simulink model "PVArrayGrid"  (R2024b)
settings: Solver=FixedStepDiscrete  StartTime=0.0  StopTime=2.5  RelTol=1e-3
PreLoadFcn:
  | Ts_Power=1e-6;
  | Ts_Control=100e-6;
InitFcn:
  | Ts_Power=1e-6;
  | Ts_Control=100e-6;
undefined symbols (not defined in the file): D1, Delta, DiscIntNeverNeededParam
libraries: spsSeriesRLCBranchLib x5, spsMeanLib x3, spsThreePhaseTransformerTwoWindingsLib x2, spsDistributedParametersLineLib x2, spsThreePhaseParallelRLCLoadLib x2, spsFourierLib x2, slpidlib x2, spsabctodq0Lib x2, spsVoltageMeasurementLib x2, spsThreePhaseSeriesRLCLoadLib x1, spsThreeLevelBridgeLib x1, spsThreePhaseSourceLib x1
(part 1 of 2)
settings Model: SimulationMode=accelerator  Creator=The MathWorks, Inc.  LastModifiedBy=chang
settings SolverCC: AlgebraicLoopSolver=TrustRegion
settings DataIOCC: LimitDataPoints=on  SaveFormat=Array  SignalLogging=off  DSMLogging=off  ReturnWorkspaceOutputs=off
settings OptimizationCC: ExpressionDepthLimit=2147483647  EfficientMapNaN2IntZero=off  LifeSpan=inf
settings DebuggingCC: UnderspecifiedInitializationDetection=Classic  MergeDetectMultiDrivingBlocksExec=none  SolverPrmCheckMsg=warning  FcnCallInpInsideContextMsg=warning  UnconnectedInputMsg=warning  UnconnectedOutputMsg=warning  UnconnectedLineMsg=warning  StateNameClashWarn=warning  SubsystemReferenceDiagnosticForUnitTest=warning  SFUnexpectedBacktrackingDiag=warning  SFNoUnconditionalDefaultTransitionDiag=warning  SFExecutionAtInitializationDiag=none  ArithmeticOperatorsInVariantConditions=warning
settings HardwareCC: ProdBitPerPointer=32  ProdBitPerSizeT=32  ProdBitPerPtrDiffT=32  ProdLargestAtomicFloat=None  ProdIntDivRoundTo=Undefined  ProdEndianess=Unspecified  ProdWordSize=32  ProdHWDeviceType=32-bit Generic  TargetBitPerPointer=64  TargetBitPerSizeT=64  TargetBitPerPtrDiffT=64  TargetLongLongMode=on  TargetIntDivRoundTo=Zero  TargetEndianess=LittleEndian  TargetWordSize=64  TargetHWDeviceType=MATLAB Host  ProdEqTarget=off
settings ModelReferenceCC: EnableRefExpFcnMdlSchedulingChecks=on  PropagateSignalLabelsOutOfModel=off
settings SFSimCC: SimUseLocalCustomCode=off  CustomCodeUndefinedFunction=UseInterfaceOnly
settings RTWCC: GPUComputeCapability=3.5
settings CodeAppCC: MaxIdLength=128
settings GRTTargetCC: TargetLangStandard=C89/C90 (ANSI)  CombineOutputUpdateFcns=off  GRTInterface=on
settings ConfigComp: CovMetricSettings=dw  CovSaveCumulativeToWorkspaceVar=on  CovSaveSingleToWorkspaceVar=on  CovExternalEMLEnable=off  CovSFcnEnable=off
settings SimscapeCC: SimscapeNormalizeSystem=off

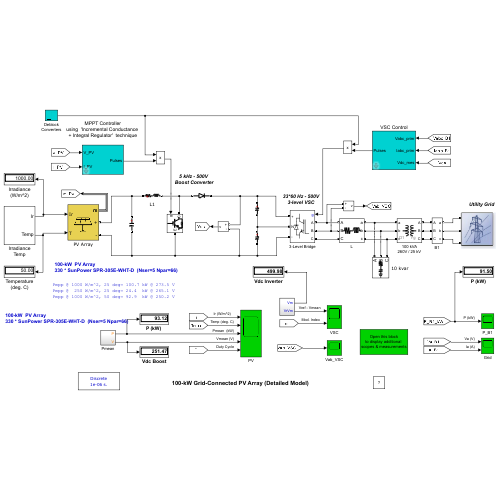
[thumbnail: Simulink's stored preview of the top-level diagram]
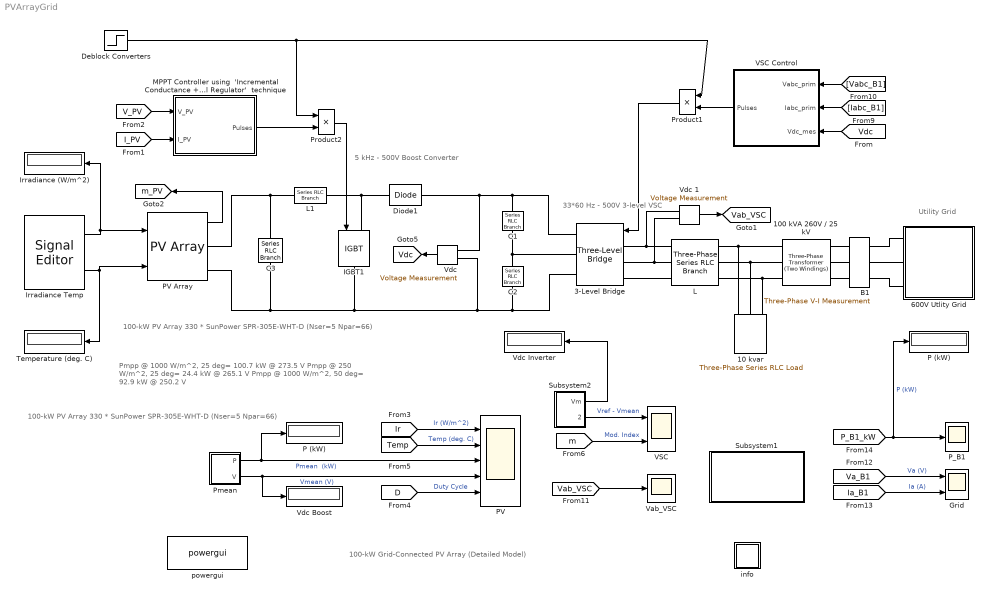
== system PVArrayGrid ==
  note: 5 kHz - 500V
      | Boost Converter
  note: 33*60 Hz - 500V
      | 3-level VSC
  note: 100-kW Grid-Connected PV Array (Detailed Model)
  note: Utility Grid
  note: Pmpp @ 1000 W/m^2, 25 deg= 100.7 kW @ 273.5 V
      | Pmpp @  250 W/m^2, 25 deg= 24.4  kW @ 265.1 V
      | Pmpp @ 1000 W/m^2, 50 deg= 92.9  kW @ 250.2 V
  note: 100-kW  PV Array
      | 330 * SunPower SPR-305E-WHT-D  (Nser=5 Npar=66)
  note: 100-kW  PV Array
      | 330 * SunPower SPR-305E-WHT-D  (Nser=5 Npar=66)
  10 kvar : spsThreePhaseSeriesRLCLoadLib/Three-Phase Series RLC Load  LConnTagsString=A|B|C  Configuration=Y (grounded)  NominalVoltage=240  Vabc=[1e3 1e3 1e3]  Vabcp=[1e3 1e3 1e3]  NominalFrequency=60  UnbalancedPower=off  ActivePower=10e3/100  InductivePower=0  CapacitivePower=10e3  Pabc=[10e3 9e3 11e3]  QLabc=[100 90 110]  QCabc=[100 90 110]  Pabcp=[10e3 9e3 11e3]  QLabcp=[100 90 110]  QCabcp=[100 90 110]  Measurements=None  LoadType=constant Z
  100 kVA 260V / 25 kV : spsThreePhaseTransformerTwoWindingsLib/Three-Phase Transformer (Two Windings)  Winding1Connection=Yg  Winding2Connection=Delta (D1)  CoreType=Three single-phase transformers  SetSaturation=off  Hysteresis=off  DataFile='hysteresis'  SetInitialFlux=off  Measurements=None  UNITS=pu  NominalPower=[100e3 , 60 ]  Winding1=[ 25e3 , 0.001 , 0.03 ]  Winding2=[ 260 , 0.001 , 0.03 ]  Rm=500  Lm=500  L0=0.5  Saturation=[ 0,0 ; 0.0024,1.2 ; 1.0,1.52 ]  InitialFluxes=[ 0.8 , -0.8 , 0.7 ]  BreakLoop=off  DiscreteSolver=Trapezoidal iterative  DataType=off  TransfoNumber=0
  3-Level Bridge : spsThreeLevelBridgeLib/Three-Level Bridge  Arms=3  SnubberResistance=1e6  SbubberCapacitance=inf  Device=IGBT / Diodes  Ron=0.2e-3  ForwardVoltages="[  0  0 ]"  Measurements=None
      settings: AttributesFormatString=\n
  600V Utlity Grid : Subsystem
      mask Display: image('$imagefile')
  B1 : spsThreePhaseVIMeasurementLib/Three-Phase V-I Measurement  VoltageMeasurement=phase-to-ground  SetLabelV=on  LabelV=Vabc_B1  Vpu=off  VpuLL=off  CurrentMeasurement=yes  SetLabelI=on  LabelI=Iabc_B1  Ipu=off  Pbase=100e6  Vbase=500e3  OutputType=Magnitude  PhasorSimulation=off  PSBequivalent=0
  C1 : spsSeriesRLCBranchLib/Series RLC Branch  LConnTagsString=__new0  RConnTagsString=__new0  BranchType=C  Resistance=1.0  Inductance=1.0  SetiL0=off  InitialCurrent=0  Capacitance=12000e-06  Setx0=off  InitialVoltage=0  Measurements=None
  C2 : spsSeriesRLCBranchLib/Series RLC Branch  LConnTagsString=__new0  RConnTagsString=__new0  BranchType=C  Resistance=1.0  Inductance=1.0  SetiL0=off  InitialCurrent=0  Capacitance=12000e-06  Setx0=off  InitialVoltage=0  Measurements=None
  C3 : spsSeriesRLCBranchLib/Series RLC Branch  LConnTagsString=__new0  RConnTagsString=__new0  BranchType=C  Resistance=1.0  Inductance=1.0  SetiL0=off  InitialCurrent=0  Capacitance=100e-6  Setx0=off  InitialVoltage=0  Measurements=Branch voltage
  Deblock Converters : Step  Time=0.05  SampleTime=0
  Diode1 : spsDiodeLib/Diode  Ron=1e-4  Lon=0  Vf=0  IC=0  UseSnubber=off  Rs=inf  Cs=inf  Measurements=off
  Grid : Scope  NumInputPorts=2
  IGBT1 : spsIGBTLib/IGBT  Ron=0.001  Lon=0  Vf=0  Tf=0  Tt=0  IC=0  Rs=1e5  Cs=inf  Measurements=off
  Irradiance (W/m^2) : Display
      settings: Format=bank  Decimation=1000
  Irradiance Temp : SignalEditorBlockLib/Signal Editor  FileName=PVArrayGridData.mat  ActiveScenario=Ramp_up_down_Irradiance  ActiveSignal=Temp  IsBus=off  OutputBusObjectStr=Bus: BusObject  SampleTime=0  OutputAfterFinalValue=Extrapolation  Unit=inherit  PreserveSignalName=on  ApplySigPropsToAllScenarios=on  ApplySigPropsToAllSignals=off
  L : spsThreePhaseSeriesRLCBranchLib/Three-Phase Series RLC Branch  LConnTagsString=A|B|C  RConnTagsString=A|B|C  BranchType=RL  Resistance=500e-6*377/50/2  Inductance=500e-6/2  Capacitance=inf  Measurements=None
  L1 : spsSeriesRLCBranchLib/Series RLC Branch  LConnTagsString=__new0  RConnTagsString=__new0  BranchType=RL  Resistance=0.005  Inductance=5e-3  SetiL0=off  InitialCurrent=0  Capacitance=1e-6  Setx0=off  InitialVoltage=0  Measurements=None
  "MPPT Controller using  'Incremental Conductance + Integral Regulator'  technique " : Subsystem  mask(Boost Control - MPPT){fc=5000, T_MPPT=200e-6, Dinit=0.5}
      mask prompts: fc "PWM switching frequency (Hz)"; T_MPPT "Time window used by MPPT control (s)"; Dinit "Initial value of duty cycle"
  P (kW) : Display
      settings: Format=bank  Decimation=2000
  "P (kW) " : Display
      settings: Format=bank  Decimation=2000
  PV : Scope  NumInputPorts=5
  PV Array : spsPVArrayLib/PV Array  Npar=66  Nser=5  PlotType=array @ 1000 W/m2 & specified temperatures  S_vec="[ 1000  250 ]"  Temp_C_vec="[0 25 50  ]"  ModuleName=SunPower SPR-305E-WHT-D  PlotWhenSelected=off  Pm=305.226  Ncell=96  Voc=64.2  Isc=5.96  Vm=54.7  Im=5.58  beta_Voc_pc=-0.2727  alpha_Isc_pc=0.061745  beta_Voc=-0.17507  alpha_Isc=0.00368  IL=5.9657  I0=6.3076e-12  nI=0.94489  Rsh=393.2054  Rs=0.37428  RobustModel=off  RobustCellTemperature=25  BAL=on  Tc=1e-6  Tfilter=5e-5
  P_B1 : Scope
  Pmean : Subsystem
  Product1 : Product  RndMeth=Zero
  Product2 : Product  RndMeth=Zero
  Subsystem1 : Subsystem
      mask Display: disp('Open this block\nto display additional \nscopes & measurements')
  Subsystem2 : Subsystem
  Temperature (deg. C) : Display
      settings: Format=bank  Decimation=1000
  VSC : Scope  NumInputPorts=2
  VSC Control : Subsystem  mask(VSC Main Controller){nom=[ 100e3  60 ], Vnom=[ 25e3 260 ], Vnom_dc=500, RLxfo=[0.002  0.06 ], RLchoke=[2e-3  250e-6  ], K_VDCreg=[7  800], K_Ireg=[0.3 20], Ts=Ts_Control}
      mask prompts: nom "Nominal power and frequency [ Pnom(VA)  Fnom(Hz) ]:"; Vnom "Nominal primary and secondary voltages (Vrms LL) [ Vnom_prim   Vnom_sec ]:"; Vnom_dc "Nominal DC bus voltage (V):"; RLxfo "Total transformer leakage impedance (pu/Pnom) [ Rxfo  Lxf ]"; RLchoke "Choke impedance [ R(ohm) L(H) ]"; K_VDCreg "VDC regultator gains [ Kp  Ki ]:"; K_Ireg "Current regulator gains [ Kp  Ki ]:"; Ts "Sample time"
      mask init:
      | Pnom=nom(1);
      | Fnom=nom(2);
      | Vnom_prim=Vnom(1);
      | Vnom_sec=Vnom(2);
      | Zbase=Vnom_sec^2/Pnom;
      | Rtot_pu=RLxfo(1) + RLchoke(1)/Zbase;
      | Ltot_pu=RLxfo(2) + RLchoke(2)/(Zbase/(2*pi*Fnom));
      | Kp_VDCreg=K_VDCreg(1);
      | Ki_VDCreg=K_VDCreg(2);
      | Kp_Ireg=K_Ireg(1);
      | Ki_Ireg=K_Ireg(2);
      | Vdc_ref=Vnom_dc;
      | % Used to determine initial value of Boost Control (MPPT)
      | assignin('base','Vdc_ref_Inv',Vdc_ref);
  Vab_VSC : Scope
  "Vdc " : spsVoltageMeasurementLib/Voltage Measurement  Tag=PoWeRsYsTeMmEaSuReMeNt  PhasorSimulation=off  OutputType=Magnitude  PSBequivalent=0
  Vdc 1 : spsVoltageMeasurementLib/Voltage Measurement  Tag=PoWeRsYsTeMmEaSuReMeNt  PhasorSimulation=off  OutputType=Magnitude  PSBequivalent=0
  Vdc Boost : Display
      settings: Format=bank  Decimation=2000
  Vdc Inverter : Display
      settings: Format=bank  Decimation=2000
  info : Subsystem
      settings: OpenFcn="showExample(\"simscapeelectricalsps/PVArrayGridExample\")"
      mask Display: disp('?')
  powergui : spspowerguiLib/powergui  Priority=1  SimulationMode=Discrete  SampleTime=Ts_Power  frequency=60  Iterations=50  frequencyindice=0  Pbase=100e6  ErrMax=1e-4  UnitsV=kV  UnitsW=MW  buscounter=0  FunctionMessages=off  echomessages=off  EnableUseOfTLC=off  CurrentSourceSwitches=off  DisableSnubberDevices=off  DisableRonSwitches=off  DisableVfSwitches=off  DisplayEquations=off  AutomaticDiscreteSolvers=off  SolverType=Tustin/Backward Euler (TBE)  Interpol=off  ExternalGateDelay=off  methode=off  Ts=0  x0status=blocks  SPID=off  SwTol=0  HookPort=off  NonlinearTolerance=1e-8  nMaxIteration=10  ContinueOnMaxIteration=off  RestoreLinks=warning  ResistiveCurrentMeasurement=off  Frange=[0:2:500]  Ylog=off  Xlog=on  ShowGrid=off  save=off  variable=ZData  structure=0  ZoomFFT=on  StartTime=0.0  cycles=1  DisplayStyle=1  fundamental=60  FreqAxis=off  MaxFrequency=1000  frequencyindicesteady=1  RmsSteady=1  display=off
  tag scope: Vab_VSC=global, Vdc=global, m_PV=global
  wires:
  "Vdc "/1 -> [Vdc]
  Product2/1 -> IGBT1/1
  "MPPT Controller using  'Incremental Conductance + Integral Regulator'  technique "/1(Pulses) -> Product2/2
  Deblock Converters/1 -> Product1/1, Product2/1
  [Vabc_B1] -> VSC Control/1(Vabc_prim)
  [Iabc_B1] -> VSC Control/2(Iabc_prim)
  [Vdc] -> VSC Control/3(Vdc_mes)
  VSC Control/1(Pulses) -> Product1/2
  Product1/1 -> 3-Level Bridge/1
  [I_PV] -> "MPPT Controller using  'Incremental Conductance + Integral Regulator'  technique "/2(I_PV)
  [V_PV] -> "MPPT Controller using  'Incremental Conductance + Integral Regulator'  technique "/1(V_PV)
  Pmean/1(P) -> "P (kW) "/1, PV/3  "Pmean  (kW)"
  [m] -> VSC/2  "Mod. Index"
  Vdc 1/1 -> [Vab_VSC]
  [Vab_VSC] -> Vab_VSC/1
  [Ia_B1] -> Grid/2  "Ia (A)"
  [Va_B1] -> Grid/1  "Va (V)"
  [P_B1_kW] -> P_B1/1, P (kW)/1  "P (kW)"
  Pmean/2(V) -> Vdc Boost/1, PV/4  "Vmean (V)"
  Subsystem2/2(VrVm) -> VSC/1  "Vref - Vmean"
  Subsystem2/1(Vm) -> Vdc Inverter/1
  PV Array/1 -> [m_PV]
  Irradiance Temp/1 -> PV Array/1, Irradiance (W/m^2)/1
  Irradiance Temp/2 -> PV Array/2, Temperature (deg. C)/1
  [D] -> PV/5  "Duty Cycle"
  [Temp] -> PV/2  "Temp (deg. C)"
  [Ir] -> PV/1  "Ir (W/m^2)"
  connections:
  3-Level Bridge/RConn1 -- Diode1/RConn1 -- "Vdc "/LConn1 -- C1/LConn1
  L1/RConn1 -- Diode1/LConn1 -- IGBT1/LConn1
  3-Level Bridge/RConn3 -- C2/RConn1 -- "Vdc "/LConn2 -- IGBT1/RConn1 -- PV Array/RConn2 -- C3/RConn1
  3-Level Bridge/LConn1 -- L/LConn1 -- Vdc 1/LConn1
  3-Level Bridge/LConn2 -- L/LConn2 -- Vdc 1/LConn2
  3-Level Bridge/LConn3 -- L/LConn3
  L/RConn1 -- 100 kVA 260V / 25 kV/RConn1 -- 10 kvar/LConn1
  L/RConn2 -- 100 kVA 260V / 25 kV/RConn2 -- 10 kvar/LConn2
  L/RConn3 -- 100 kVA 260V / 25 kV/RConn3 -- 10 kvar/LConn3
  B1/LConn1 -- 100 kVA 260V / 25 kV/LConn1
  B1/LConn2 -- 100 kVA 260V / 25 kV/LConn2
  B1/LConn3 -- 100 kVA 260V / 25 kV/LConn3
  C2/LConn1 -- C1/RConn1 -- 3-Level Bridge/RConn2
  C3/LConn1 -- PV Array/RConn1 -- L1/LConn1
  B1/RConn2 -- 600V Utlity Grid/LConn2
  B1/RConn1 -- 600V Utlity Grid/LConn1
  B1/RConn3 -- 600V Utlity Grid/LConn3

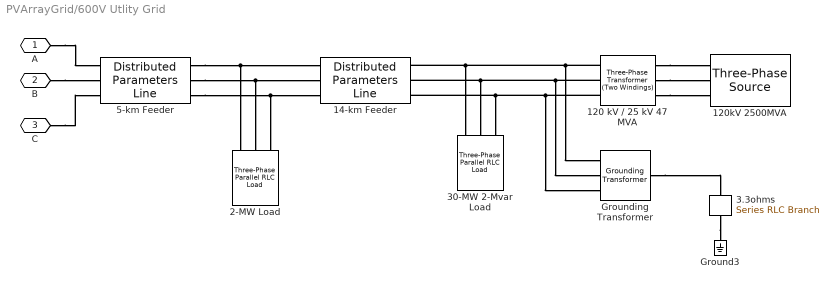
== system PVArrayGrid/600V Utlity Grid ==
  120 kV / 25 kV 47 MVA : spsThreePhaseTransformerTwoWindingsLib/Three-Phase Transformer (Two Windings)  Winding1Connection=Yg  Winding2Connection=Delta (D1)  CoreType=Three single-phase transformers  SetSaturation=off  Hysteresis=off  DataFile='basic_model'  SetInitialFlux=off  Measurements=None  UNITS=pu  NominalPower=[47e6 60 ]  Winding1="[ 120e3  0.08/30   0.08 ]"  Winding2="[ 25e3  0.08/30  0.08]"  Rm=500  Lm=500  L0=0.5  Saturation="[ 0,0  ;  0.005,1.2  ;  1.0,1.4 ]"  InitialFluxes=[ 0.8 , -0.8 , 0.7 ]  BreakLoop=off  DiscreteSolver=Trapezoidal iterative  DataType=off  TransfoNumber=0
  120kV 2500MVA : spsThreePhaseSourceLib/Three-Phase Source  InternalConnection=Yg  VoltagePhases=off  Voltage=120e3  PhaseAngle=0  Voltage_phases=[25e3 25e3 25e3]/sqrt(3)  PhaseAngles_phases=[0 -120 +120]  Frequency=60  NonIdealSource=on  SpecifyImpedance=on  Resistance=0.8929  Inductance=16.58e-3  ShortCircuitLevel=2500e6  BaseVoltage=120e3  XRratio=7  BusType=swing  Pref=0  Qref=0  Prefabc=[10e3, 10e3, 10e3]  Qrefabc=[0, 0, 0]  Qmin=-inf  Qmax=inf
  14-km Feeder : spsDistributedParametersLineLib/Distributed Parameters Line  Phases=3  Length=14  Frequency=60  Resistance=[0.1153 0.413]  Inductance=[1.05e-3 3.32e-3]  Capacitance=[11.33e-009 5.01e-009]  x1=[-5.8e-05 -2.72104735733765e-09 0 0;-5.7e-05 -2.72148457100924e-09 0 0;-5.6e-05 -2.72192139789718e-09 0 0;-5.5e-05 -2.72235783793939e-09 0 0;-5.4e-05 -2.72279389107383e-09 0 0;-5.3e-05 -2.72322955723854e-09 0 0;-5.2e-05 -2.7236648363716e-09 0 0;-5.1e-05 -2.72409972841114e-09 0 0;-5e-05 -2.72453423329536e-09 0 0;-4.9e-05 -2.7249683509625e-09 -3790.73535189766 -24061.4134200297;-4.8e-05 -2.72540208135087e-09 -3781.66414358226 -24062.8407837241;-4.7e-05 -2.72583542439882e-09 -3772.59239780806 -24064.2647275522;-4.6e-05 -2.72626838004477e-09 -3763.52011586433 -24065.6852513116;-4.5e-05 -2.72670094822718e-09 -3754.44729904047 -24067.1023548004;-4.4e-05 -2.72713312888457e-09 -3745.37394862591 -24068.5160378172;-4.3e-05 -2.72756492195553e-09 -3736.30006591019 -24069.9263001612;-4.2e-05 -2.72799632737868e-09 -3727.2256521829 -24071.3331416318;-4.1e-05 -2.72842734509272e-09 -3718.15070873373 -24072.7365620291;-4e-05 -2.72885797503638e-09 -3709.07523685241 -24074.1365611537;-3.9e-05 -2.72928821714846e-09 -3699.99923782879 -24075.5331388067;-3.8e-05 -2.72971807136783e-09 -3690.92271295276 -24076.9262947894;-3.7e-05 -2.73014753763337e-09 -3681.8456635143 -24078.3160289039;-3.6e-05 -2.73057661588407e-09 -3672.76809080346 -24079.7023409528;-3.5e-05 -2.73100530605893e-09 -3663.68999611036 -24081.0852307389;-3.4e-05 -2.73143360809703e-09 -3654.61138072521 -24082.4646980658;-3.3e-05 -2.7318615219375e-09 -3645.53224593827 -24083.8407427373;-3.2e-05 -2.73228904751952e-09 -3636.45259303991 -24085.213364558;-3.1e-05 -2.73271618478233e-09 -3627.37242332053 -24086.5825633327;-3e-05 -2.73314293366523e-09 -3618.29173807063 -24087.9483388669;-2.9e-05 -2.73356929410757e-09 -3609.21053858078 -24089.3106909664;-2.8e-05 -2.73399526604874e-09 -3600.12882614163 -24090.6696194376;-2.7e-05 -2.73442084942822e-09 -3591.04660204388 -24092.0251240874;-2.6e-05 -2.73484604418551e-09 -3581.96386757832 -24093.3772047232;-2.5e-05 -2.73527085026018e-09 -3572.88062403581 -24094.7258611527;-2.4e-05 -2.73569526759187e-09 -3563.79687270728 -24096.0710931843;-2.3e-05 -2.73611929612025e-09 -3554.71261488374 -24097.4129006268;-2.2e-05 -2.73654293578505e-09 -3545.62785185626 -24098.7512832896;-2.1e-05 -2.73696618652608e-09 -3536.54258491599 -24100.0862409823;-2e-05 -2.73738904828317e-09 -3527.45681535414 -24101.4177735154;-1.9e-05 -2.73781152099623e-09 -3518.37054446202 -24102.7458806994;-1.8e-05 -2.73823360460521e-09 -3509.28377353097 -24104.0705623458;-1.7e-05 -2.73865529905013e-09 -3500.19650385244 -24105.3918182661;-1.6e-05 -2.73907660427106e-09 -3491.10873671792 -24106.7096482727;-1.5e-05 -2.73949752020812e-09 -3482.020473419 -24108.0240521782;-1.4e-05 -2.73991804680148e-09 -3472.93171524731 -24109.3350297958;-1.3e-05 -2.74033818399138e-09 -3463.84246349457 -24110.6425809393;-1.2e-05 -2.74075793171812e-09 -3454.75271945257 -24111.9467054227;-1.1e-05 -2.74117728992202e-09 -3445.66248441316 -24113.2474030608;-1e-05 -2.74159625854351e-09 -3436.57175966826 -24114.5446736687;-9e-06 -2.74201483752302e-09 -3427.48054650988 -24115.8385170619;-8e-06 -2.74243302680107e-09 -3418.38884623008 -24117.1289330567;-7e-06 -2.74285082631822e-09 -3409.29666012098 -24118.4159214696;-6e-06 -2.74326823601511e-09 -3400.20398947479 -24119.6994821177;-5e-06 -2.7436852558324e-09 -3391.11083558379 -24120.9796148187;-4e-06 -2.74410188571082e-09 -3382.01719974031 -24122.2563193904;-3e-06 -2.74451812559117e-09 -3372.92308323676 -24123.5295956516;-2e-06 -2.74493397541429e-09 -3363.82848736562 -24124.7994434213;-1e-06 -2.74534943512107e-09 -3354.73341341943 -24126.0658625189]  x2=[-5.8e-05 -2.96070926633097e-09 0 0;-5.7e-05 -2.96113943631565e-09 0 0;-5.6e-05 -2.96156918545639e-09 0 0;-5.5e-05 -2.96199851369209e-09 0 0;-5.4e-05 -2.96242742096175e-09 0 0;-5.3e-05 -2.9628559072044e-09 0 0;-5.2e-05 -2.96328397235915e-09 0 0;-5.1e-05 -2.96371161636516e-09 0 0;-5e-05 -2.96413883916166e-09 0 0;-4.9e-05 -2.96456564068792e-09 -3379.39242591109 -24244.0512732198;-4.8e-05 -2.96499202088329e-09 -3370.25239397928 -24245.3235513097;-4.7e-05 -2.96541797968717e-09 -3361.11188305945 -24246.5923835984;-4.6e-05 -2.96584351703902e-09 -3351.97089445066 -24247.8577699056;-4.5e-05 -2.96626863287837e-09 -3342.82942945205 -24249.1197100514;-4.4e-05 -2.96669332714479e-09 -3333.68748936283 -24250.3782038566;-4.3e-05 -2.96711759977792e-09 -3324.54507548227 -24251.6332511421;-4.2e-05 -2.96754145071747e-09 -3315.40218910971 -24252.8848517298;-4.1e-05 -2.9679648799032e-09 -3306.25883154456 -24254.1330054416;-4e-05 -2.96838788727493e-09 -3297.1150040863 -24255.3777121002;-3.9e-05 -2.96881047277254e-09 -3287.97070803446 -24256.6189715286;-3.8e-05 -2.96923263633598e-09 -3278.82594468866 -24257.8567835506;-3.7e-05 -2.96965437790523e-09 -3269.68071534857 -24259.0911479901;-3.6e-05 -2.97007569742038e-09 -3260.53502131393 -24260.3220646718;-3.5e-05 -2.97049659482152e-09 -3251.38886388455 -24261.5495334206;-3.4e-05 -2.97091707004886e-09 -3242.24224436029 -24262.7735540622;-3.3e-05 -2.97133712304262e-09 -3233.09516404111 -24263.9941264226;-3.2e-05 -2.97175675374311e-09 -3223.947624227 -24265.2112503283;-3.1e-05 -2.97217596209069e-09 -3214.79962621804 -24266.4249256063;-3e-05 -2.97259474802578e-09 -3205.65117131435 -24267.6351520841;-2.9e-05 -2.97301311148887e-09 -3196.50226081614 -24268.8419295897;-2.8e-05 -2.97343105242049e-09 -3187.35289602367 -24270.0452579517;-2.7e-05 -2.97384857076124e-09 -3178.20307823727 -24271.245136999;-2.6e-05 -2.97426566645179e-09 -3169.05280875733 -24272.4415665611;-2.5e-05 -2.97468233943286e-09 -3159.90208888432 -24273.6345464679;-2.4e-05 -2.97509858964522e-09 -3150.75091991874 -24274.8240765499;-2.3e-05 -2.97551441702973e-09 -3141.5993031612 -24276.010156638;-2.2e-05 -2.97592982152728e-09 -3132.44723991233 -24277.1927865637;-2.1e-05 -2.97634480307883e-09 -3123.29473147284 -24278.3719661589;-2e-05 -2.97675936162541e-09 -3114.14177914353 -24279.547695256;-1.9e-05 -2.9771734971081e-09 -3104.98838422521 -24280.7199736878;-1.8e-05 -2.97758720946803e-09 -3095.8345480188 -24281.8888012879;-1.7e-05 -2.97800049864642e-09 -3086.68027182526 -24283.05417789;-1.6e-05 -2.97841336458453e-09 -3077.52555694561 -24284.2161033286;-1.5e-05 -2.97882580722367e-09 -3068.37040468094 -24285.3745774385;-1.4e-05 -2.97923782650523e-09 -3059.21481633242 -24286.529600055;-1.3e-05 -2.97964942237066e-09 -3050.05879320124 -24287.6811710141;-1.2e-05 -2.98006059476145e-09 -3040.90233658868 -24288.829290152;-1.1e-05 -2.98047134361916e-09 -3031.74544779609 -24289.9739573056;-1e-05 -2.98088166888544e-09 -3022.58812812485 -24291.1151723122;-9e-06 -2.98129157050194e-09 -3013.43037887644 -24292.2529350096;-8e-06 -2.98170104841043e-09 -3004.27220135236 -24293.387245236;-7e-06 -2.9821101025527e-09 -2995.1135968542 -24294.5181028304;-6e-06 -2.98251873287062e-09 -2985.9545666836 -24295.645507632;-5e-06 -2.98292693930612e-09 -2976.79511214227 -24296.7694594805;-4e-06 -2.98333472180117e-09 -2967.63523453196 -24297.8899582161;-3e-06 -2.98374208029782e-09 -2958.4749351545 -24299.0070036798;-2e-06 -2.98414901473818e-09 -2949.31421531178 -24300.1205957126;-1e-06 -2.98455552506442e-09 -2940.15307630573 -24301.2307341564]  x3=[-5.8e-05 -8.55897584940559e-12 0 0;-5.7e-05 -8.56403370536508e-12 0 0;-5.6e-05 -8.5690903441844e-12 0 0;-5.5e-05 -8.57414576514486e-12 0 0;-5.4e-05 -8.579199967528e-12 0 0;-5.3e-05 -8.5842529506155e-12 0 0;-5.2e-05 -8.5893047136892e-12 0 0;-5.1e-05 -8.59435525603115e-12 0 0;-5e-05 -8.59940457692354e-12 0 0;-4.9e-05 -8.60445267564877e-12 -23.544284738252 -155.681477773854;-4.8e-05 -8.60949955148938e-12 -23.4855925321333 -155.690342696974;-4.7e-05 -8.61454520372809e-12 -23.4268969881881 -155.699185493025;-4.6e-05 -8.61958963164782e-12 -23.3681981147585 -155.70800616075;-4.5e-05 -8.62463283453162e-12 -23.3094959201867 -155.716804698894;-4.4e-05 -8.62967481166275e-12 -23.2507904128157 -155.725581106208;-4.3e-05 -8.63471556232464e-12 -23.1920816009888 -155.734335381443;-4.2e-05 -8.63975508580088e-12 -23.13336949305 -155.743067523356;-4.1e-05 -8.64479338137524e-12 -23.0746540973434 -155.751777530706;-4e-05 -8.64983044833166e-12 -23.0159354222139 -155.760465402255;-3.9e-05 -8.65486628595427e-12 -22.9572134760066 -155.769131136768;-3.8e-05 -8.65990089352737e-12 -22.8984882670674 -155.777774733014;-3.7e-05 -8.66493427033542e-12 -22.8397598037422 -155.786396189764;-3.6e-05 -8.66996641566306e-12 -22.7810280943779 -155.794995505792;-3.5e-05 -8.67499732879512e-12 -22.7222931473214 -155.803572679878;-3.4e-05 -8.6800270090166e-12 -22.6635549709203 -155.8121277108;-3.3e-05 -8.68505545561266e-12 -22.6048135735226 -155.820660597345;-3.2e-05 -8.69008266786864e-12 -22.5460689634767 -155.829171338299;-3.1e-05 -8.69510864507008e-12 -22.4873211491317 -155.837659932452;-3e-05 -8.70013338650266e-12 -22.4285701388368 -155.846126378598;-2.9e-05 -8.70515689145226e-12 -22.3698159409419 -155.854570675534;-2.8e-05 -8.71017915920492e-12 -22.3110585637972 -155.86299282206;-2.7e-05 -8.71520018904688e-12 -22.2522980157536 -155.871392816978;-2.6e-05 -8.72021998026452e-12 -22.1935343051622 -155.879770659096;-2.5e-05 -8.72523853214443e-12 -22.1347674403745 -155.888126347221;-2.4e-05 -8.73025584397336e-12 -22.0759974297428 -155.896459880168;-2.3e-05 -8.73527191503823e-12 -22.0172242816195 -155.90477125675;-2.2e-05 -8.74028674462615e-12 -21.9584480043576 -155.913060475788;-2.1e-05 -8.74530033202441e-12 -21.8996686063106 -155.921327536102;-2e-05 -8.75031267652044e-12 -21.8408860958322 -155.929572436519;-1.9e-05 -8.7553237774019e-12 -21.7821004812769 -155.937795175866;-1.8e-05 -8.7603336339566e-12 -21.7233117709993 -155.945995752974;-1.7e-05 -8.76534224547251e-12 -21.6645199733546 -155.954174166679;-1.6e-05 -8.77034961123781e-12 -21.6057250966984 -155.962330415817;-1.5e-05 -8.77535573054084e-12 -21.5469271493869 -155.97046449923;-1.4e-05 -8.78036060267011e-12 -21.4881261397765 -155.978576415762;-1.3e-05 -8.78536422691433e-12 -21.4293220762242 -155.98666616426;-1.2e-05 -8.79036660256235e-12 -21.3705149670873 -155.994733743573;-1.1e-05 -8.79536772890325e-12 -21.3117048207236 -156.002779152556;-1e-05 -8.80036760522623e-12 -21.2528916454914 -156.010802390064;-9e-06 -8.80536623082072e-12 -21.1940754497493 -156.018803454959;-8e-06 -8.81036360497629e-12 -21.1352562418564 -156.026782346102;-7e-06 -8.81535972698271e-12 -21.0764340301722 -156.034739062359;-6e-06 -8.82035459612991e-12 -21.0176088230567 -156.0426736026;-5e-06 -8.82534821170802e-12 -20.9587806288703 -156.050585965698;-4e-06 -8.83034057300732e-12 -20.8999494559738 -156.058476150526;-3e-06 -8.8353316793183e-12 -20.8411153127283 -156.066344155965;-2e-06 -8.84032152993161e-12 -20.7822782074955 -156.074189980896;-1e-06 -8.84531012413806e-12 -20.7234381486375 -156.082013624204]  x4=[-5.8e-05 1.93112949511814e-12 0 0;-5.7e-05 1.93533782185214e-12 0 0;-5.6e-05 1.93954587353147e-12 0 0;-5.5e-05 1.94375364955807e-12 0 0;-5.4e-05 1.94796114933393e-12 0 0;-5.3e-05 1.95216837226107e-12 0 0;-5.2e-05 1.95637531774154e-12 0 0;-5.1e-05 1.96058198517746e-12 0 0;-5e-05 1.96478837397095e-12 0 0;-4.9e-05 1.96899448352419e-12 -1.35581366009174 -2.15298522698201;-4.8e-05 1.9732003132394e-12 -1.3550019074566 -2.1534962036844;-4.7e-05 1.97740586251885e-12 -1.35418996224548 -2.15400687432695;-4.6e-05 1.98161113076482e-12 -1.35337782457375 -2.15451723883709;-4.5e-05 1.98581611737966e-12 -1.35256549455686 -2.15502729714228;-4.4e-05 1.99002082176574e-12 -1.35175297231025 -2.15553704917003;-4.3e-05 1.99422524332548e-12 -1.35094025794939 -2.15604649484789;-4.2e-05 1.99842938146134e-12 -1.35012735158979 -2.15655563410346;-4.1e-05 2.00263323557581e-12 -1.34931425334699 -2.15706446686438;-4e-05 2.00683680507144e-12 -1.34850096333653 -2.15757299305833;-3.9e-05 2.01104008935081e-12 -1.34768748167402 -2.15808121261305;-3.8e-05 2.01524308781652e-12 -1.34687380847506 -2.15858912545629;-3.7e-05 2.01944579987126e-12 -1.3460599438553 -2.15909673151588;-3.6e-05 2.0236482249177e-12 -1.3452458879304 -2.15960403071968;-3.5e-05 2.02785036235861e-12 -1.34443164081605 -2.16011102299557;-3.4e-05 2.03205221159675e-12 -1.34361720262799 -2.16061770827152;-3.3e-05 2.03625377203495e-12 -1.34280257348195 -2.1611240864755;-3.2e-05 2.04045504307608e-12 -1.34198775349373 -2.16163015753556;-3.1e-05 2.04465602412305e-12 -1.34117274277912 -2.16213592137976;-3e-05 2.04885671457879e-12 -1.34035754145394 -2.16264137793623;-2.9e-05 2.0530571138463e-12 -1.33954214963407 -2.16314652713313;-2.8e-05 2.05725722132861e-12 -1.33872656743539 -2.16365136889866;-2.7e-05 2.06145703642879e-12 -1.33791079497381 -2.16415590316108;-2.6e-05 2.06565655854995e-12 -1.33709483236526 -2.16466012984869;-2.5e-05 2.06985578709525e-12 -1.33627867972572 -2.16516404888981;-2.4e-05 2.07405472146787e-12 -1.33546233717118 -2.16566766021284;-2.3e-05 2.07825336107107e-12 -1.33464580481765 -2.16617096374619;-2.2e-05 2.08245170530811e-12 -1.33382908278119 -2.16667395941834;-2.1e-05 2.08664975358233e-12 -1.33301217117788 -2.1671766471578;-2e-05 2.09084750529707e-12 -1.3321950701238 -2.16767902689313;-1.9e-05 2.09504495985576e-12 -1.3313777797351 -2.16818109855292;-1.8e-05 2.09924211666184e-12 -1.33056030012792 -2.16868286206583;-1.7e-05 2.10343897511879e-12 -1.32974263141845 -2.16918431736053;-1.6e-05 2.10763553463016e-12 -1.32892477372289 -2.16968546436577;-1.5e-05 2.11183179459951e-12 -1.32810672715749 -2.17018630301031;-1.4e-05 2.11602775443047e-12 -1.3272884918385 -2.17068683322299;-1.3e-05 2.1202234135267e-12 -1.32647006788222 -2.17118705493265;-1.2e-05 2.12441877129189e-12 -1.32565145540496 -2.17168696806821;-1.1e-05 2.12861382712979e-12 -1.32483265452306 -2.17218657255863;-1e-05 2.1328085804442e-12 -1.32401366535289 -2.17268586833288;-9e-06 2.13700303063895e-12 -1.32319448801086 -2.17318485532002;-8e-06 2.1411971771179e-12 -1.32237512261338 -2.17368353344913;-7e-06 2.14539101928499e-12 -1.3215555692769 -2.17418190264933;-6e-06 2.14958455654416e-12 -1.3207358281179 -2.17467996284979;-5e-06 2.15377778829943e-12 -1.31991589925289 -2.17517771397973;-4e-06 2.15797071395484e-12 -1.3190957827984 -2.17567515596841;-3e-06 2.16216333291449e-12 -1.31827547887097 -2.17617228874513;-2e-06 2.16635564458251e-12 -1.3174549875872 -2.17666911223923;-1e-06 2.17054764836308e-12 -1.31663430906369 -2.17716562638011]  x5=5.70973484498186e-05  V1=[0 0 0 2.868e-09 2.436e+04 2.436e+04;0 0 0 377 377 377;1.571 1.571 1.571 -0.5389 -0.156 -1.727]  V2=[0 0 0 2.996e-09 2.448e+04 2.448e+04;0 0 0 377 377 377;1.571 1.571 1.571 -0.5232 -0.1382 -1.709]  I1=[0 0 0 1.022e-11 157.5 157.5;0 0 0 377 377 377;1.571 1.571 1.571 -1.198 -0.1498 -1.721]  I2=[0 0 0 6.231e-12 2.544 2.544;0 0 0 377 377 377;1.571 1.571 1.571 1.184 -0.5617 -2.133]  nHarmo=2  Measurements=None  Decoupling=off  VsMag0=0  VrMag0=0  VsAngle0=0  VrAngle0=0  IsMag0=0  IrMag0=0  IsAngle0=0  IrAngle0=0
  2-MW Load : spsThreePhaseParallelRLCLoadLib/Three-Phase Parallel RLC Load  LConnTagsString=A|B|C  Configuration=Y (grounded)  NominalVoltage=25e3  Vabc=[1e3 1e3 1e3]  Vabcp=[1e3 1e3 1e3]  NominalFrequency=60  UnbalancedPower=off  ActivePower=2e6  InductivePower=0  CapacitivePower=0  Pabc=[10e3 9e3 11e3]  QLabc=[100 90 110]  QCabc=[100 90 110]  Pabcp=[10e3 9e3 11e3]  QLabcp=[100 90 110]  QCabcp=[100 90 110]  Measurements=None  LoadType=constant Z
  "3.3ohms " : spsSeriesRLCBranchLib/Series RLC Branch  LConnTagsString=__new0  RConnTagsString=__new0  BranchType=R  Resistance=3.3  Inductance=[]  SetiL0=off  InitialCurrent=0  Capacitance=[]  Setx0=off  InitialVoltage=0  Measurements=None
  30-MW 2-Mvar Load : spsThreePhaseParallelRLCLoadLib/Three-Phase Parallel RLC Load  LConnTagsString=A|B|C  Configuration=Y (grounded)  NominalVoltage=25e3  Vabc=[1e3 1e3 1e3]  Vabcp=[1e3 1e3 1e3]  NominalFrequency=60  UnbalancedPower=off  ActivePower=30e6  InductivePower=2e6  CapacitivePower=0  Pabc=[10e3 9e3 11e3]  QLabc=[100 90 110]  QCabc=[100 90 110]  Pabcp=[10e3 9e3 11e3]  QLabcp=[100 90 110]  QCabcp=[100 90 110]  Measurements=None  LoadType=constant Z
  5-km Feeder : spsDistributedParametersLineLib/Distributed Parameters Line  Phases=3  Length=5  Frequency=60  Resistance=[0.1153 0.413]  Inductance=[1.05e-3 3.32e-3]  Capacitance=[11.33e-009 5.01e-009]  x1=[-2.1e-05 -2.68978914771068e-09 -3537.17773129423 -24101.4118174736;-2e-05 -2.6902063858996e-09 -3528.0914619567 -24102.743589357;-1.9e-05 -2.6906232417502e-09 -3519.00469119869 -24104.0719357029;-1.8e-05 -2.69103971520323e-09 -3509.91742031163 -24105.3968563227;-1.7e-05 -2.6914558061995e-09 -3500.82965058704 -24106.718351028;-1.6e-05 -2.69187151467987e-09 -3491.74138331647 -24108.036419631;-1.5e-05 -2.69228684058527e-09 -3482.65261979158 -24109.3510619444;-1.4e-05 -2.69270178385667e-09 -3473.56336130409 -24110.6622777813;-1.3e-05 -2.69311634443509e-09 -3464.47360914577 -24111.9700669554;-1.2e-05 -2.69353052226162e-09 -3455.38336460849 -24113.2744292808;-1.1e-05 -2.69394431727739e-09 -3446.29262898418 -24114.5753645721;-1e-05 -2.69435772942359e-09 -3437.20140356482 -24115.8728726445;-9e-06 -2.69477075864148e-09 -3428.10968964249 -24117.1669533136;-8e-06 -2.69518340487234e-09 -3419.01748850932 -24118.4576063953;-7e-06 -2.69559566805753e-09 -3409.92480145752 -24119.7448317063;-6e-06 -2.69600754813846e-09 -3400.83162977935 -24121.0286290637;-5e-06 -2.69641904505659e-09 -3391.73797476717 -24122.308998285;-4e-06 -2.69683015875344e-09 -3382.64383771337 -24123.5859391882;-3e-06 -2.69724088917058e-09 -3373.54921991045 -24124.8594515919;-2e-06 -2.69765123624964e-09 -3364.45412265095 -24126.129535315;-1e-06 -2.69806119993229e-09 -3355.35854722748 -24127.396190177]  x2=[-2.1e-05 -2.73605852038205e-09 -3536.54258491599 -24100.0862409823;-2e-05 -2.73648129377405e-09 -3527.45681535414 -24101.4177735154;-1.9e-05 -2.73690367825103e-09 -3518.37054446202 -24102.7458806994;-1.8e-05 -2.73732567375297e-09 -3509.28377353097 -24104.0705623458;-1.7e-05 -2.73774728021987e-09 -3500.19650385244 -24105.3918182661;-1.6e-05 -2.73816849759183e-09 -3491.10873671792 -24106.7096482727;-1.5e-05 -2.73858932580899e-09 -3482.020473419 -24108.0240521782;-1.4e-05 -2.73900976481152e-09 -3472.93171524731 -24109.3350297958;-1.3e-05 -2.73942981453968e-09 -3463.84246349457 -24110.6425809393;-1.2e-05 -2.73984947493378e-09 -3454.75271945257 -24111.9467054227;-1.1e-05 -2.74026874593415e-09 -3445.66248441316 -24113.2474030608;-1e-05 -2.74068762748123e-09 -3436.57175966826 -24114.5446736687;-9e-06 -2.74110611951547e-09 -3427.48054650988 -24115.8385170619;-8e-06 -2.74152422197741e-09 -3418.38884623008 -24117.1289330567;-7e-06 -2.7419419348076e-09 -3409.29666012098 -24118.4159214696;-6e-06 -2.74235925794671e-09 -3400.20398947479 -24119.6994821177;-5e-06 -2.7427761913354e-09 -3391.11083558379 -24120.9796148187;-4e-06 -2.74319273491442e-09 -3382.01719974031 -24122.2563193904;-3e-06 -2.74360888862458e-09 -3372.92308323676 -24123.5295956516;-2e-06 -2.74402465240673e-09 -3363.82848736562 -24124.7994434213;-1e-06 -2.74444002620178e-09 -3354.73341341943 -24126.0658625189]  x3=[-2.1e-05 -4.98188152304993e-12 -11.1569792961309 -79.1361755515201;-2e-05 -4.98525864556532e-12 -11.1271448686803 -79.140376010016;-1.9e-05 -4.98863505956428e-12 -11.0973088598142 -79.1445652208994;-1.8e-05 -4.99201076456694e-12 -11.0674712737731 -79.148743183575;-1.7e-05 -4.99538576009355e-12 -11.0376321147975 -79.1529098974491;-1.6e-05 -4.99876004566443e-12 -11.0077913871281 -79.1570653619295;-1.5e-05 -5.00213362080002e-12 -10.9779490950062 -79.1612095764255;-1.4e-05 -5.00550648502088e-12 -10.9481052426728 -79.1653425403482;-1.3e-05 -5.00887863784763e-12 -10.9182598343696 -79.1694642531102;-1.2e-05 -5.01225007880101e-12 -10.8884128743381 -79.1735747141257;-1.1e-05 -5.01562080740188e-12 -10.8585643668203 -79.1776739228106;-1e-05 -5.01899082317118e-12 -10.8287143160584 -79.1817618785822;-9e-06 -5.02236012562995e-12 -10.7988627262946 -79.1858385808596;-8e-06 -5.02572871429934e-12 -10.7690096017716 -79.1899040290633;-7e-06 -5.0290965887006e-12 -10.7391549467322 -79.1939582226155;-6e-06 -5.03246374835507e-12 -10.7092987654194 -79.1980011609402;-5e-06 -5.03583019278421e-12 -10.6794410620764 -79.2020328434627;-4e-06 -5.03919592150958e-12 -10.6495818409466 -79.2060532696099;-3e-06 -5.04256093405282e-12 -10.6197211062738 -79.2100624388105;-2e-06 -5.04592522993569e-12 -10.5898588623017 -79.2140603504948;-1e-06 -5.04928880868006e-12 -10.5599951132746 -79.2180470040944]  x4=[-2.1e-05 -3.51860546156375e-12 -12.5606324025953 -78.9000787577201;-2e-05 -3.5166409547337e-12 -12.5308868817917 -78.9048083977352;-1.9e-05 -3.51467594811054e-12 -12.5011395800696 -78.9095268236173;-1.8e-05 -3.51271044197356e-12 -12.4713905016568 -78.9142340346958;-1.7e-05 -3.51074443660207e-12 -12.4416396507813 -78.9189300303018;-1.6e-05 -3.50877793227551e-12 -12.4118870316713 -78.9236148097677;-1.5e-05 -3.50681092927335e-12 -12.3821326485554 -78.9282883724279;-1.4e-05 -3.50484342787515e-12 -12.3523765056622 -78.9329507176181;-1.3e-05 -3.50287542836054e-12 -12.3226186072209 -78.9376018446756;-1.2e-05 -3.5009069310092e-12 -12.2928589574607 -78.9422417529395;-1.1e-05 -3.49893793610092e-12 -12.263097560611 -78.9468704417502;-1e-05 -3.49696844391552e-12 -12.2333344209017 -78.9514879104501;-9e-06 -3.49499845473292e-12 -12.2035695425628 -78.9560941583827;-8e-06 -3.49302796883309e-12 -12.1738029298245 -78.9606891848935;-7e-06 -3.49105698649609e-12 -12.1440345869173 -78.9652729893294;-6e-06 -3.48908550800204e-12 -12.1142645180719 -78.969845571039;-5e-06 -3.48711353363112e-12 -12.0844927275194 -78.9744069293723;-4e-06 -3.4851410636636e-12 -12.0547192194909 -78.9789570636812;-3e-06 -3.48316809837981e-12 -12.024943998218 -78.9834959733189;-2e-06 -3.48119463806015e-12 -11.9951670679324 -78.9880236576404;-1e-06 -3.4792206829851e-12 -11.965388432866 -78.9925401160021]  x5=2.03919101606495e-05  V1=[0 0 0 2.827e-09 2.436e+04 2.436e+04;0 0 0 377 377 377;1.571 1.571 1.571 -0.5179 -0.1443 -1.715]  V2=[0 0 0 2.868e-09 2.436e+04 2.436e+04;0 0 0 377 377 377;1.571 1.571 1.571 -0.5251 -0.1443 -1.715]  I1=[0 0 0 7.018e-12 79.92 79.92;0 0 0 377 377 377;1.571 1.571 1.571 -1.622 -0.1386 -1.709]  I2=[0 0 0 7.946e-12 79.89 79.89;0 0 0 377 377 377;1.571 1.571 1.571 0.3547 -0.1565 -1.727]  nHarmo=2  Measurements=None  Decoupling=off  VsMag0=0  VrMag0=0  VsAngle0=0  VrAngle0=0  IsMag0=0  IrMag0=0  IsAngle0=0  IrAngle0=0
  Ground3 : spsGroundLib/Ground  LConnTagsString=a
  "Grounding Transformer " : spsGroundingTransformerLib/Grounding Transformer   UNITS=pu  NominalPower="[100e6   60]"  NominalVoltage=25e3  ZeroSequenceImpedance_pu=[0.025 0.75]  MagnetizationBranch_pu=[500 500]  ZeroSequenceImpedance_SI=[0.052083 589.05]  MagnetizationBranch_SI=[1041.7 3.927e+005]  Measurements=None
  A : PMIOPort  Side=Left
  B : PMIOPort  Port=2  Side=Left
  C : PMIOPort  Port=3  Side=Left
  connections:
  "3.3ohms "/RConn1 -- Ground3/LConn1
  120 kV / 25 kV 47 MVA/LConn1 -- 120kV 2500MVA/RConn1
  120 kV / 25 kV 47 MVA/LConn2 -- 120kV 2500MVA/RConn2
  120 kV / 25 kV 47 MVA/LConn3 -- 120kV 2500MVA/RConn3
  120 kV / 25 kV 47 MVA/RConn1 -- "Grounding Transformer "/LConn1 -- 14-km Feeder/RConn1 -- 30-MW 2-Mvar Load/LConn1
  120 kV / 25 kV 47 MVA/RConn2 -- "Grounding Transformer "/LConn2 -- 14-km Feeder/RConn2 -- 30-MW 2-Mvar Load/LConn2
  120 kV / 25 kV 47 MVA/RConn3 -- "Grounding Transformer "/LConn3 -- 14-km Feeder/RConn3 -- 30-MW 2-Mvar Load/LConn3
  5-km Feeder/RConn1 -- 14-km Feeder/LConn1 -- 2-MW Load/LConn1
  5-km Feeder/RConn2 -- 14-km Feeder/LConn2 -- 2-MW Load/LConn2
  5-km Feeder/RConn3 -- 14-km Feeder/LConn3 -- 2-MW Load/LConn3
  A/RConn1 -- 5-km Feeder/LConn1
  B/RConn1 -- 5-km Feeder/LConn2
  C/RConn1 -- 5-km Feeder/LConn3
  "Grounding Transformer "/RConn1 -- "3.3ohms "/LConn1

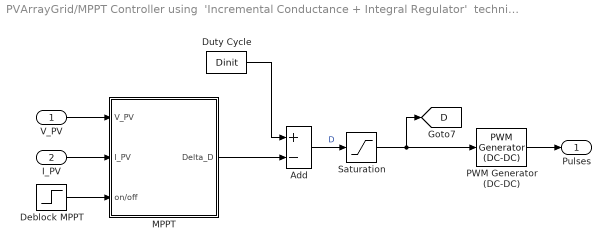
== system PVArrayGrid/MPPT Controller using  'Incremental Conductance + Integral Regulator'  technique  ==
  V_PV : Inport
  I_PV : Inport  Port=2
  Add : Sum  Inputs=+-
  Deblock MPPT : Step  Time=0.4  SampleTime=0
  Duty Cycle : Constant  Value=Dinit
  MPPT : Subsystem
  PWM Generator (DC-DC) : spsPWMGeneratorDCDCLib/PWM Generator (DC-DC)  Fsw=fc  Ts=Ts_Power
  Saturation : Saturate  UpperLimit=1  LowerLimit=0
  Pulses : Outport  VectorParamsAs1DForOutWhenUnconnected=off
  tag scope: D=global
  wires:
  V_PV/1 -> MPPT/1(V_PV)
  I_PV/1 -> MPPT/2(I_PV)
  PWM Generator (DC-DC)/1 -> Pulses/1
  Deblock MPPT/1 -> MPPT/3(on/off)
  Saturation/1 -> PWM Generator (DC-DC)/1, [D]
  Add/1 -> Saturation/1  "D"
  MPPT/1(Delta_D) -> Add/2
  Duty Cycle/1 -> Add/1

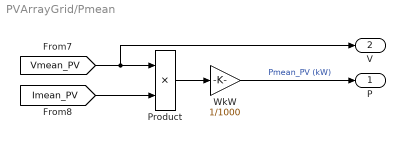
== system PVArrayGrid/Pmean ==
  Product : Product  RndMeth=Zero
  WkW : Gain  Gain=1/1000
  P : Outport  VectorParamsAs1DForOutWhenUnconnected=off
  V : Outport  Port=2  VectorParamsAs1DForOutWhenUnconnected=off
  wires:
  [Vmean_PV] -> Product/1, V/1
  Product/1 -> WkW/1
  [Imean_PV] -> Product/2
  WkW/1 -> P/1  "Pmean_PV (kW)"

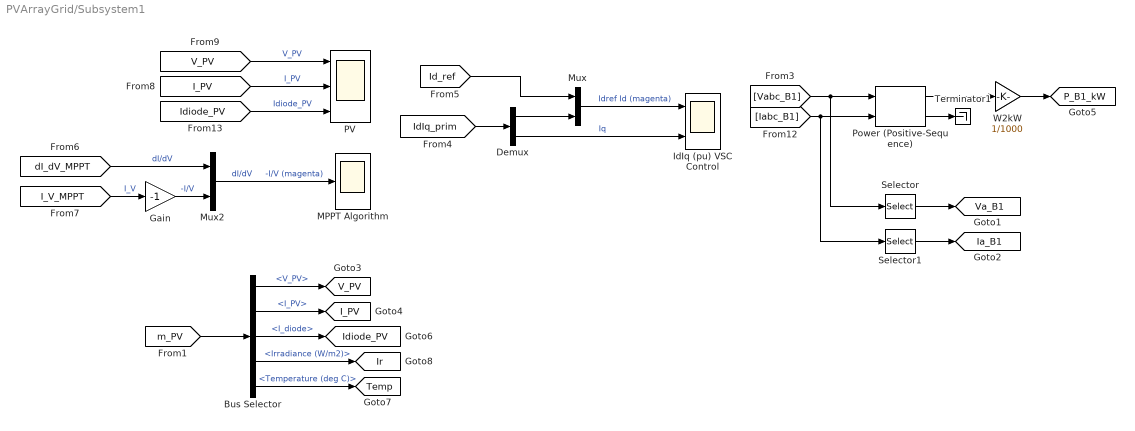
== system PVArrayGrid/Subsystem1 ==
  Bus Selector : BusSelector  OutputSignals=V_PV,I_PV,I_diode,Irradiance (W/m2),Temperature (deg C)
  Demux : Demux  Outputs=2
  Gain : Gain  Gain=-1
  IdIq (pu) VSC Control : Scope  NumInputPorts=2
  MPPT Algorithm : Scope
  Mux : Mux  Inputs=2
  Mux2 : Mux  Inputs=2
  PV : Scope  NumInputPorts=3
  Power (Positive-Sequence) : spsPowerPositiveSequenceLib/Power (Positive-Sequence)  Freq=60  Vinit=[0, 0]  Iinit=[0, 0]  Ts=Ts_Control
  Selector : Selector  InputPortWidth=3  IndexOptions=Index vector (dialog)  Indices=[1]  OutputSizes=1
  Selector1 : Selector  InputPortWidth=3  IndexOptions=Index vector (dialog)  Indices=[1]  OutputSizes=1
  Terminator1 : Terminator
  W2kW : Gain  Gain=1/1000
  tag scope: I_PV=global, Ia_B1=global, Idiode_PV=global, Ir=global, P_B1_kW=global, Temp=global, V_PV=global, Va_B1=global
  wires:
  [Vabc_B1] -> Power (Positive-Sequence)/1, Selector/1
  [Iabc_B1] -> Power (Positive-Sequence)/2, Selector1/1
  Power (Positive-Sequence)/1 -> W2kW/1
  [I_V_MPPT] -> Gain/1  "I_V"
  [IdIq_prim] -> Demux/1
  [Id_ref] -> Mux/1
  Demux/1 -> Mux/2
  Mux/1 -> IdIq (pu) VSC Control/1  "Idref Id (magenta)"
  Demux/2 -> IdIq (pu) VSC Control/2  "Iq"
  Selector/1 -> [Va_B1]
  Selector1/1 -> [Ia_B1]
  [V_PV] -> PV/1  "V_PV"
  [I_PV] -> PV/2  "I_PV"
  [Idiode_PV] -> PV/3  "Idiode_PV"
  [dI_dV_MPPT] -> Mux2/1  "dI/dV"
  Gain/1 -> Mux2/2  "-I/V"
  Mux2/1 -> MPPT Algorithm/1  "dI/dV     -I/V (magenta)"
  W2kW/1 -> [P_B1_kW]
  [m_PV] -> Bus Selector/1
  Bus Selector/1 -> [V_PV]  "<V_PV>"
  Bus Selector/2 -> [I_PV]  "<I_PV>"
  Bus Selector/4 -> [Ir]  "<Irradiance (W/m2)>"
  Bus Selector/3 -> [Idiode_PV]  "<I_diode>"
  Bus Selector/5 -> [Temp]  "<Temperature (deg C)>"
  Power (Positive-Sequence)/2 -> Terminator1/1

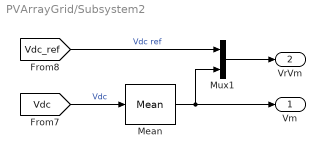
== system PVArrayGrid/Subsystem2 ==
  Mean : spsMeanLib/Mean  Freq=60  Vinit=0  Ts=Ts_Control
  Mux1 : Mux  Inputs=2
  Vm : Outport  VectorParamsAs1DForOutWhenUnconnected=off
  VrVm : Outport  Port=2  VectorParamsAs1DForOutWhenUnconnected=off
  wires:
  [Vdc_ref] -> Mux1/1  "Vdc ref"
  [Vdc] -> Mean/1  "Vdc"
  Mux1/1 -> VrVm/1
  Mean/1 -> Mux1/2, Vm/1

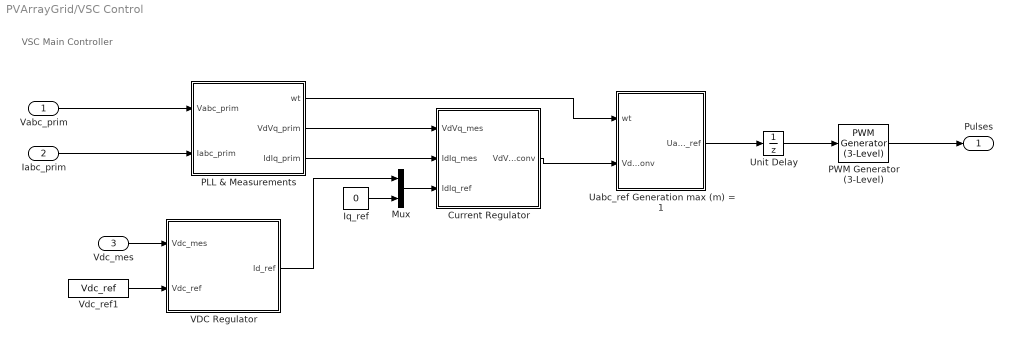
== system PVArrayGrid/VSC Control ==
  note: VSC Main Controller
  Vabc_prim : Inport  PortDimensions=3
  Iabc_prim : Inport  Port=2  PortDimensions=3
  Vdc_mes : Inport  Port=3  PortDimensions=1
  Current Regulator : Subsystem
  Iq_ref : Constant  Value=0
  Mux : Mux  Inputs=2
  PLL & Measurements : Subsystem
  PWM Generator (3-Level) : spsPWMGenerator3LevelLib/PWM Generator (3-Level)  ModulatorType=Three-phase bridge (12 pulses)  ModulatorMode=Unsynchronized  nF=27  Fc=33*60  ModulatingSignals=off  m=0.8  Freq=60  Phase=0  Ts=Ts_Power
  Uabc_ref Generation max (m) = 1 : Subsystem
  Unit Delay : UnitDelay  SampleTime=Ts_Control  HasFrameUpgradeWarning=on
  VDC Regulator : Subsystem
  Vdc_ref1 : Constant  Value=Vdc_ref
  Pulses : Outport  VectorParamsAs1DForOutWhenUnconnected=off
  wires:
  VDC Regulator/1(Id_ref) -> Mux/1
  PLL & Measurements/1(wt) -> Uabc_ref Generation max (m) = 1/1(wt)
  Current Regulator/1(VdVq_conv) -> Uabc_ref Generation max (m) = 1/2(VdVq_conv)
  Iq_ref/1 -> Mux/2
  Mux/1 -> Current Regulator/3(IdIq_ref)
  PLL & Measurements/3(IdIq_prim) -> Current Regulator/2(IdIq_mes)
  PLL & Measurements/2(VdVq_prim) -> Current Regulator/1(VdVq_mes)
  Vdc_mes/1 -> VDC Regulator/1(Vdc_mes)
  Vabc_prim/1 -> PLL & Measurements/1(Vabc_prim)
  Iabc_prim/1 -> PLL & Measurements/2(Iabc_prim)
  Unit Delay/1 -> PWM Generator (3-Level)/1
  PWM Generator (3-Level)/1 -> Pulses/1
  Uabc_ref Generation max (m) = 1/1(Uabc_ref) -> Unit Delay/1
  Vdc_ref1/1 -> VDC Regulator/2(Vdc_ref)

== system PVArrayGrid/info ==

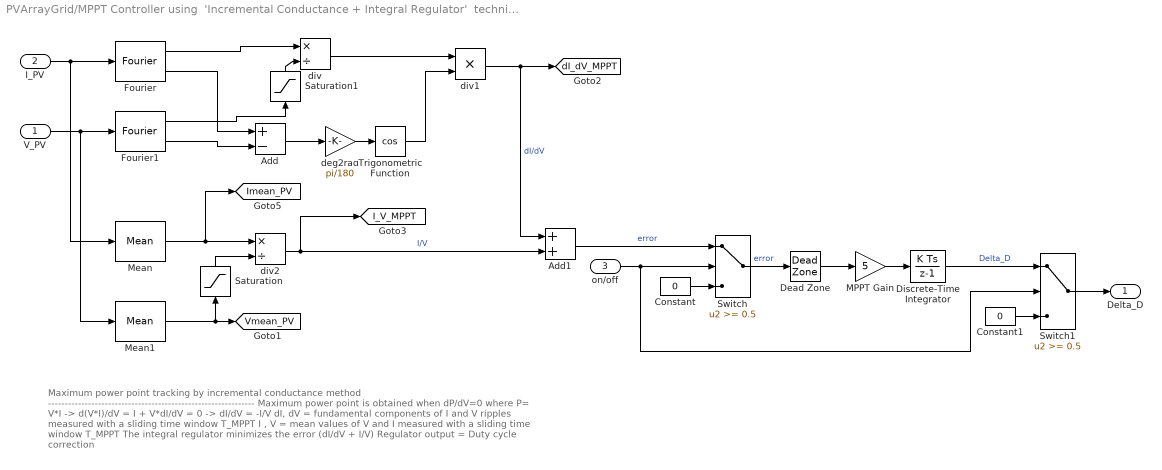
== system PVArrayGrid/MPPT Controller using  'Incremental Conductance + Integral Regulator'  technique /MPPT ==
  note: Maximum power point tracking by incremental conductance method
      | --------------------------------------------------------------
      | Maximum power point is obtained when dP/dV=0  where P= V*I
      | -> d(V*I)/dV = I + V*dI/dV = 0
      | -> dI/dV = -I/V
      |
      | dI, dV  = fundamental components of I and V ripples measured with a sliding time window T_MPPT
      | I , V   = mean values of V and I measured with a sliding time window T_MPPT
      |
      | The integral regulator minimizes the error (dI/dV + I/V)
      | Regulator output = Duty cycle correction
  V_PV : Inport
  I_PV : Inport  Port=2
  on/off : Inport  Port=3
  Add : Sum  Inputs=+-
  Add1 : Sum
  Constant : Constant  Value=0
  Constant1 : Constant  Value=0
  Dead Zone : DeadZone  LowerValue=-0.05  UpperValue=0.05
  Discrete-Time Integrator : DiscreteIntegrator  SampleTime=Ts_Control  LimitOutput=on  UpperSaturationLimit=1  LowerSaturationLimit=-1  ICPrevOutput=DiscIntNeverNeededParam  ICPrevScaledInput=DiscIntNeverNeededParam
  Fourier : spsFourierLib/Fourier  Freq=1/T_MPPT  n=1  InInit=[0, 0]  Ts=Ts_Control
  Fourier1 : spsFourierLib/Fourier  Freq=1/T_MPPT  n=1  InInit=[0, 0]  Ts=Ts_Control
  MPPT Gain : Gain  Gain=5
  Mean : spsMeanLib/Mean  Freq=1/T_MPPT  Vinit=0  Ts=Ts_Control
  Mean1 : spsMeanLib/Mean  Freq=1/T_MPPT  Vinit=0  Ts=Ts_Control
  Saturation : Saturate  UpperLimit=inf  LowerLimit=eps
  Saturation1 : Saturate  UpperLimit=inf  LowerLimit=eps
  Switch : Switch  Threshold=0.5  SaturateOnIntegerOverflow=off  InputSameDT=off
  Switch1 : Switch  Threshold=0.5  SaturateOnIntegerOverflow=off  InputSameDT=off
  Trigonometric Function : Trigonometry  Operator=cos
  deg2rad : Gain  Gain=pi/180
  div : Product  Inputs=*/  RndMeth=Zero
  div1 : Product  Inputs=**  RndMeth=Zero
  div2 : Product  Inputs=*/  RndMeth=Zero
  Delta_D : Outport  VectorParamsAs1DForOutWhenUnconnected=off
  tag scope: I_V_MPPT=global, Imean_PV=global, Vmean_PV=global, dI_dV_MPPT=global
  wires:
  Dead Zone/1 -> MPPT Gain/1
  Switch/1 -> Dead Zone/1  "error"
  Saturation1/1 -> div/2
  Saturation/1 -> div2/2
  Switch1/1 -> Delta_D/1
  on/off/1 -> Switch/2, Switch1/2
  Constant1/1 -> Switch1/3
  Discrete-Time Integrator/1 -> Switch1/1  "Delta_D"
  Constant/1 -> Switch/3
  MPPT Gain/1 -> Discrete-Time Integrator/1
  Add1/1 -> Switch/1  "error"
  div2/1 -> Add1/2, [I_V_MPPT]  "I/V"
  Mean1/1 -> Saturation/1, [Vmean_PV]
  Mean/1 -> div2/1, [Imean_PV]
  div1/1 -> Add1/1, [dI_dV_MPPT]  "dI/dV"
  Trigonometric Function/1 -> div1/2
  div/1 -> div1/1
  deg2rad/1 -> Trigonometric Function/1
  Add/1 -> deg2rad/1
  Fourier1/1 -> Saturation1/1
  Fourier1/2 -> Add/2
  Fourier/2 -> Add/1
  V_PV/1 -> Mean1/1, Fourier1/1
  I_PV/1 -> Mean/1, Fourier/1
  Fourier/1 -> div/1
